simulink model "exercise02"  (R2022a)
settings: Solver=VariableStepAuto  StartTime=0.0  StopTime=10.0  RelTol=1e-3
settings Model: Creator=ac133867  LastModifiedBy=cunis
settings DebuggingCC: UnconnectedInputMsg=warning  UnconnectedOutputMsg=warning  UnconnectedLineMsg=warning
settings RTWCC: DLArmComputeVersion=19.05

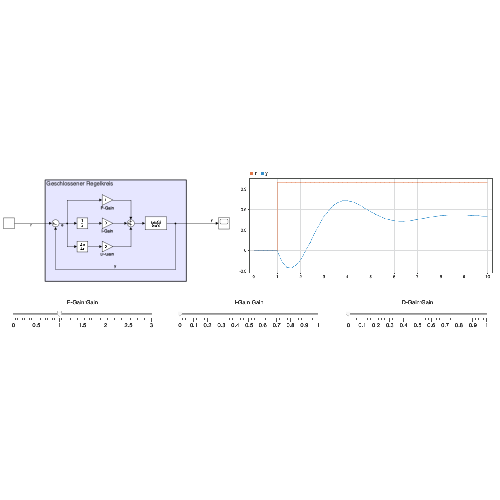
[thumbnail: Simulink's stored preview of the top-level diagram]
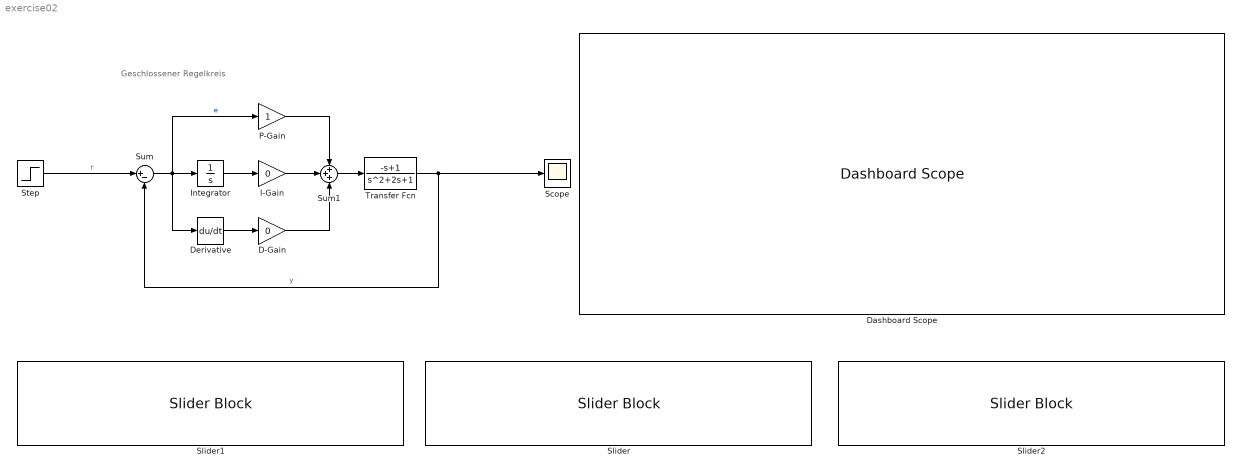
== system exercise02 ==
  note: Geschlossener Regelkreis
  D-Gain : Gain  Gain=0
  Dashboard Scope : DashboardScope
  Derivative : Derivative
  I-Gain : Gain  Gain=0
  Integrator : Integrator
  P-Gain : Gain
  Scope : Scope
  Slider : SliderBlock  ScaleMax=1
  Slider1 : SliderBlock  ScaleMax=3  TickInterval=.5
  Slider2 : SliderBlock  ScaleMax=1
  Step : Step  SampleTime=0
  Sum : Sum  Inputs=|+-
  Sum1 : Sum  Inputs=+++
  Transfer Fcn : TransferFcn  Numerator=[-1 1]
  wires:
  Step/1 -> Sum/1  "r"
  Sum1/1 -> Transfer Fcn/1
  Sum/1 -> Derivative/1, P-Gain/1, Integrator/1  "e"
  Transfer Fcn/1 -> Scope/1, Sum/2  "y"
  P-Gain/1 -> Sum1/1
  Integrator/1 -> I-Gain/1
  I-Gain/1 -> Sum1/2
  Derivative/1 -> D-Gain/1
  D-Gain/1 -> Sum1/3
